simulink model "neuromodels"  (Simulink 2.20)
settings: Solver=ode45  StartTime=0.0  StopTime=999999  MaxStep=10  RelTol=1e-3  AbsTol=1e-3
values from neighbouring files (symbols this model uses):
  a = a    [buttfilt.m]
settings Model: SaveTime=off  SaveOutput=off  ConsistencyChecking=off  RTWPlaceOutputsASAP=off

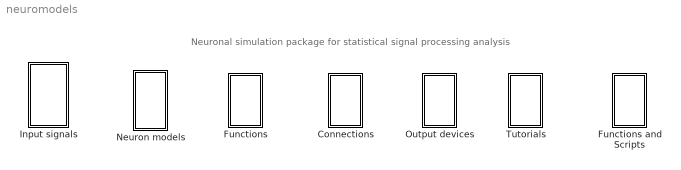
== system neuromodels ==
  note: Neuronal simulation package for statistical signal processing analysis
  Connections : Subsystem
  Functions : Subsystem
  Functions and Scripts : Subsystem
  "Input signals " : Subsystem
  Neuron models : Subsystem
  Output devices : Subsystem
  Tutorials : Subsystem

== system neuromodels/Connections ==
  note: Connection elements
  Gain : Gain  Gain=1
  Inner Product : Subsystem
      mask Type: Dot Product
      mask Description:
      | Inner (dot) product.
      | y=sum(u1.*u2)
      mask Help: Computes the inner (dot) product of the inputs: sum(u1.*u2).  The inputs are vectors of the same length. Output is a scalar.
      mask Display: disp('.\n')
  Sum : Sum  Inputs=++

== system neuromodels/Functions ==
  note: Functions
  Exponential  low-pass filter : DiscreteFilter  Numerator=k2  Denominator=1  SampleTime=dt  mask(Exponential low-pass filter){@1=20, @2=512, @3=tstep}
      mask prompts: @1 "Time constant [msec]"; @2 "Number of  points"; @3 "time step [msec]"
      mask help: Parameters
      mask init:
      | tau = @1; n = @2; dt = @3; t = [0:1:n-1]*dt; k2 = exp(-t/tau) ; k2 = k2/norm(k2);
      mask Display: plot(t,k2);
  Half-wave rectifier : Fcn  Expr=0.5*(u[1] + abs(u[1]))  mask(half-wave rectifier){}
      mask init:
      | x = [-2:0.1:2]; y = 0.5*(x+abs(x));
      mask Display: plot(x,y);
  LGN transfer function : DiscreteFilter  Numerator=k2  Denominator=1  SampleTime=dt  mask(LGN transfer function){@1=5.5, @2=tstep, @3=1500}
      mask prompts: @1 "cut-off frequency [Hz]"; @2 "time step [msec]"; @3 "time constant [msec]"
      mask help: Parameters
      mask init:
      | omega_c = @1*2*pi; dt = @2; tau = @3*1e-3; b = sqrt(omega_c^2 + tau^(-2)) ; tv = [0:dt:512]; tv_s = tv*1e-3; k2 = tv_s.*(tau + 0.5*(1-tau*b)*tv_s).*exp(-b*tv_s); k2 = k2/norm(k2);
      mask Display: plot(tv,k2);

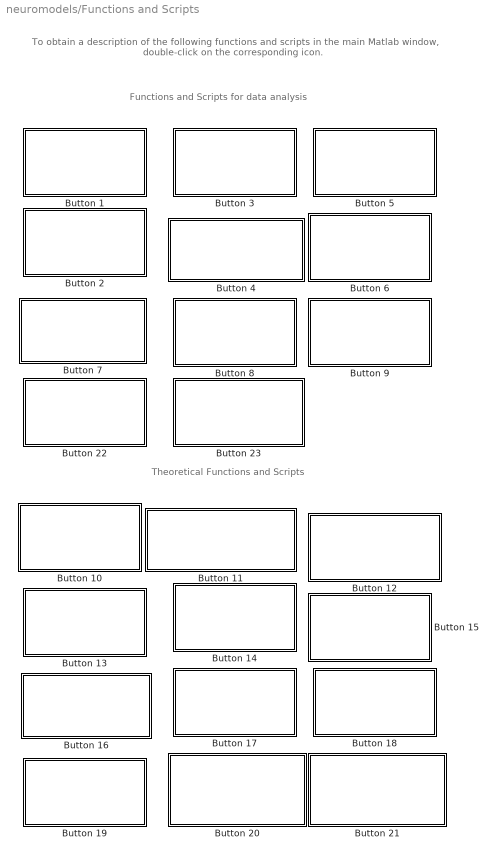
== system neuromodels/Functions and Scripts ==
  note: Functions and Scripts for data analysis
  note: To obtain a description of the following functions and scripts in
      | the main Matlab window, double-click on the corresponding icon.
  note: Theoretical Functions and Scripts
  Button 1 : Subsystem
      settings: OpenFcn=help psautostim
      mask Description: Button 1disp('End');
      mask Display: disp('Power spectrum \nand autocorrelation \nof a stimulus')
  Button 10 : Subsystem
      settings: OpenFcn=help fithifref
      mask Description: Button 10disp('End');
      mask Display: disp('F-I curve of an\nintegrate-and-fire\nneuron  ')
  Button 11 : Subsystem
      settings: OpenFcn=help fithlifref
      mask Description: Button 11disp('End');
      mask Display: disp('F-I curve of a\nleaky integrate-and-fire\nneuron ')
  Button 12 : Subsystem
      settings: OpenFcn=help gfitheor
      mask Description: Button 12disp('End');
      mask Display: disp('ISI distribution of\n random threshold \nneuron models\n(gamma and Poisson \ndistributions)  ')
  Button 13 : Subsystem
      settings: OpenFcn=help gpstheor
      mask Description: Button 13disp('End');
      mask Display: disp('Power spectrum and\nautocorrelation of\nrandom threshold\nneurons ')
  Button 14 : Subsystem
      settings: OpenFcn=help buttfilt
      mask Description: Button 14disp('End');
      mask Display: disp('Transfer function\nof a Butterworth\ndigital filter ')
  Button 15 : Subsystem
      settings: OpenFcn=help lgnfilt
      mask Description: Button 15disp('End');
      mask Display: disp('Transfer function of \na LGN thalamic\nrelay cell  ')
  Button 16 : Subsystem
      settings: OpenFcn=help poisscnt
      mask Description: Button 16disp('End');
      mask Display: disp('Count distribution for \na Poisson process ')
  Button 17 : Subsystem
      settings: OpenFcn=help neymtacnt
      mask Description: Button 17disp('End');
      mask Display: disp('Neyman type A\ncount distribution')
  Button 18 : Subsystem
      settings: OpenFcn=help prefdisp
      mask Description: Button 18disp('End');
      mask Display: disp('Variance vs. mean\ndispersion for\na Poisson process\nwith ref. period')
  Button 19 : Subsystem
      settings: OpenFcn=help sndpdisp
      mask Description: Button 19disp('End');
      mask Display: disp('Variance vs. mean\ndispersion for a\nshot noise driven\nPoisson process')
  Button 2 : Subsystem
      settings: OpenFcn=help psautospk
      mask Description: Button 2disp('End');
      mask Display: disp('Power spectrum \nand autocorrelation \nof a spike train')
  Button 20 : Subsystem
      settings: OpenFcn=help gaussroc
      mask Description: Button 20disp('End');
      mask Display: disp('ROC curves\nfor\nGaussian distributions')
  Button 21 : Subsystem
      settings: OpenFcn=help stesttheor
      mask Description: Button 21disp('End');
      mask Display: disp('Coding fraction vs. \nmean firing rate \nplot for  \nPoisson neurons')
  Button 22 : Subsystem
      settings: OpenFcn=help roc
      mask Description: Button 22disp('End');
      mask Display: disp('ROC curve \nfor two spike \ncount distributions')
  Button 23 : Subsystem
      settings: OpenFcn=help stestf
      mask Description: Button 23disp('End'); eval('help stestf1'); disp('End');
      mask Display: disp('Dependence of the \n accuracy of stimulus\n estimation on the\n mean firing rate')
  Button 3 : Subsystem
      settings: OpenFcn=help isidist
      mask Description: Button 3disp('End');
      mask Display: disp('ISI distribution\nof a spike train')
  Button 4 : Subsystem
      settings: OpenFcn=help stimest
      mask Description: Button 4disp('End');
      mask Display: disp('Estimation of a random\nstimulus from\na spike train\n(Wiener-Kolmogorov)')
  Button 5 : Subsystem
      settings: OpenFcn=help wiener1
      mask Description: Button 5disp('End');
      mask Display: disp('First order\nwiener kernel')
  Button 6 : Subsystem
      settings: OpenFcn=help countprob
      mask Description: Button 6disp('End');
      mask Display: disp('Distribution of  spike\ncounts in an\ninterval')
  Button 7 : Subsystem
      settings: OpenFcn=help dispersion
      mask Description: Button 7disp('End');
      mask Display: disp('Dispersion of the \nspike count\n(variance vs. mean)  ')
  Button 8 : Subsystem
      settings: OpenFcn=help roc
      mask Description: Button 8disp('End');
      mask Display: disp('ROC curve for\nspike count\ndistributions')
  Button 9 : Subsystem
      settings: OpenFcn=help ficurve
      mask Description: Button 9disp('End');
      mask Display: disp('Firing frequency vs. \ninjected current')

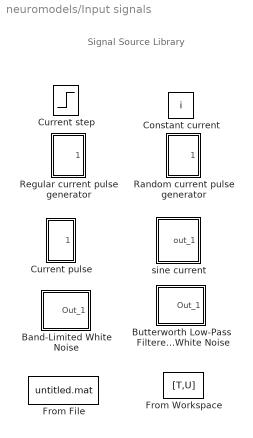
== system neuromodels/Input signals  ==
  note: Signal Source Library
  Band-Limited White Noise : Subsystem  mask(Discrete time white noise. ){@1=tstep, @2=0.1, @3=[23341]}
      mask prompts: @1 "time step [msec]"; @2 "standard deviation [nA]"; @3 "random seed"
      mask help: Discrete time white noise
      mask init:
      | dt = @1; sigma = @2; seed = @3; r = rand(1,12); r2 = [r(1),r;r,r(12)]; t =[1:13;1:13];
      mask Help: Generates a sequence of normally distributed random numbers with standard deviation sigma
      mask Display: plot(t(:),r2(:))
  Butterworth Low-Pass  Filtered White Noise : Subsystem  mask(Low-pass filtered white noise. ){@1=tstep, @2=0.63, @3=[23341], @4=240, @5=4}
      mask prompts: @1 "time step [msec]"; @2 "standard deviation [nA]"; @3 "random seed"; @4 "Cut-off frequency [Hz]"; @5 "filter order"
      mask help: Discrete time white noise
      mask init:
      | dt = @1; sigma = @2; seed = @3;[bint, a] = butter(@5,@4*2*@1*1e-3); h = freqz(bint,a); nfac = sum(h.*conj(h))/length(h); b = bint/sqrt(nfac); n = @5; x = rand(1,10*@5); y = filter(b,a,x);
      mask Help: Generates a Gaussian noise with fixed standard deviation  in the time domain and fixed cut-off frequency in the frequency domain.
      mask Display: plot((5*n:10*n),y(5*n:10*n));
  Constant current : Constant  Value=i  mask(constant current){@1=0.6}
      mask prompts: @1 "constant current value [nA]"
      mask help: Parameter
      mask init:
      | i = @1;
      mask Help: Provides a constant input current
  Current pulse : Subsystem  mask(Current step){@1=tstep, @2=100, @3=200, @4=1}
      mask prompts: @1 "time step [msec]"; @2 "start time [msec]"; @3 "pulse length [msec]"; @4 "current value [nA]"
      mask help: Parameters:
      mask init:
      | dt = @1; s = @2; w = @3; h =@4;
      mask Help: At onset tiFor a detailed description of the block, please type 'help stepc' in the main matlab window
      mask Display: plot(0,0,100,100,[10,30,30,70,70,90],[20,20,80,80,20,20])
  Current step : Step  Time=t_on  Before=i_in  After=i_fin  mask(Current step){@1=0, @2=0, @3=0}
      mask prompts: @1 "onset time [msec]"; @2 "initial current [nA]"; @3 "final current [nA]"
      mask help: Parameters
      mask init:
      | t_on = @1; i_in = @2; i_fin = @3;
      mask Help: At onset time the value of the current switches between the initial and final value
  From Workspace : FromWorkspace  VariableName=[T,U]
  From File : FromFile  FileName=untitled.mat
  Random current pulse generator : Subsystem  mask(Pulse generator){@1=tstep, @2=100, @3=20, @4=2, @5=1}
      mask prompts: @1 "time step [msec]"; @2 "start time [msec]"; @3 "period [msec]"; @4 "width [msec]"; @5 "pulse height [nA]"
      mask help: Parameters:
      mask init:
      | dt = @1; s = @2; p = @3; w = @4; h = @5;
      mask Help: Pulse generator, for a detailled description of the model, type 'help pulsegen' in the main matlab window
      mask Display: plot(0,0,100,100,[90,75,75,60,60,35,35,20,20,10],[20,20,80,80,20,20,80,80,20,20])
  Regular current pulse generator : Subsystem  mask(Pulse generator){@1=tstep, @2=100, @3=50, @4=10, @5=1}
      mask prompts: @1 "time step [msec]"; @2 "start time [msec]"; @3 "period [msec]"; @4 "width [msec]"; @5 "pulse height [nA]"
      mask help: Parameters:
      mask init:
      | dt = @1; s = @2; p = @3; w = @4; h = @5;
      mask Help: Pulse generator, for a detailled description of the model, type 'help pulsegen' in the main matlab window
      mask Display: plot(0,0,100,100,[90,75,75,60,60,35,35,20,20,10],[20,20,80,80,20,20,80,80,20,20])
  sine current : Subsystem  mask(sine current){@1=tstep, @2=2, @3=10, @4=0.25, @5=2}
      mask prompts: @1 "time step [msec]"; @2 "sine amplitude [nA]"; @3 "frequency [Hz]"; @4 "phase [percent of period]"; @5 "offset current [nA]"
      mask help: Parameters
      mask init:
      | dt = @1; a = @2; f = @3; p = @4; o = @5;
      mask Help: For detailed information about this block, please type 'help sinec' in the main matlab window
      mask Display: plot(0,-1.2,120,1.2,(0:100),sin((2*pi).*(0:100)./100))

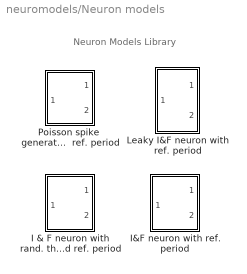
== system neuromodels/Neuron models ==
  note: Neuron Models Library
  I & F neuron with rand. thres. and ref. period : Subsystem  mask(I&F g. thres., ref. per.){@1=tstep, @2=10, @3=2, @4=0.5, @5=5}
      mask prompts: @1 "time step [msec]"; @2 "mean threshold [mV]"; @3 "gamma distr. order"; @4 "Capacitance [nF]"; @5 "refractory period [msec]"
      mask help: Parameters
      mask init:
      | dt = @1; thres = @2; n = @3; C = @4; ref = @5; if (ref<dt) disp(' '); disp('Warning: refractory period cannot be smaller than time step.'); disp(' '); end;
      mask Help: For a detailled description of the model, please type 'help giandfr' in the main matlab window
      mask Display: disp('Vm \n\n spikes')
  I&F neuron with ref. period : Subsystem  mask(I&F ref. per. ){@1=tstep, @2=10, @3=.5, @4=5}
      mask prompts: @1 "time step [msec]"; @2 "threshold [mV]"; @3 "Capacitance [nF]"; @4 "refractory period [msec]"
      mask help: Parameters
      mask init:
      | dt = @1; thres = @2; C = @3; ref = @4; if (ref<dt) disp(' '); disp('Warning: refractory period cannot be smaller than time step.'); disp(' '); end;
      mask Help: For a detailled description of the model, please type 'help iandfr' in the main matlab window
      mask Display: disp('Vm \n\n spikes')
  Leaky I&F neuron with ref. period : Subsystem  mask(L I&F ref. per.){@1=tstep, @2=10, @3=.5, @4=50, @5=5}
      mask prompts: @1 "time step [msec]"; @2 "threshold [mV]"; @3 "Capacitance [nF]"; @4 "Resistance [MOhms]"; @5 "refractory period [msec]"
      mask help: Parameters
      mask init:
      | dt = @1; thres = @2; C = @3; R = @4; ref = @5; if (ref<dt) disp(' '); disp('Warning: refractory period cannot be smaller than time step.'); disp(' '); end;
      mask Help: For a detailled description of the model, please type 'help liandfr' in the main matlab window.
      mask Display: disp('Vm \n\n spikes')
  Poisson spike  generator with  ref. period : Subsystem  mask(I&F p. thres., ref. per.){@1=tstep, @2=10, @3=.5, @4=5}
      mask prompts: @1 "time step [msec]"; @2 "mean threshold [mV]"; @3 "Capacitance [nF]"; @4 "refractory period [msec]"
      mask help: Parameters
      mask init:
      | dt = @1; thres = @2; C = @3; ref = @4; if (ref<dt) disp(' '); disp('Warning: refractory period cannot be smaller than time step.'); disp(' '); end;
      mask Help: For a detailled description of the model, please type 'help piandfr' in the main matlab window
      mask Display: disp('Vm \n\n spikes')

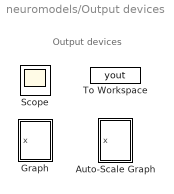
== system neuromodels/Output devices ==
  note: Output devices
  Auto-Scale Graph : Subsystem  mask(Storage scope.){@1=5, @2=-10, @3=10, @4=200, @5='y-/g--/c-./w:/m*/ro/b+'}
      mask prompts: @1 "Initial Time Range:"; @2 "Initial y-min:"; @3 "Initial y-max:"; @4 "Storage pts.:"; @5 "Line type (rgbw-.:xo):"
      mask help:
      | Storage scope using MATLAB graph window.
      | Enter plotting ranges and line type.
      mask init:
      | npts = @4; color = @5; ax = [0, @1, @2, @3]; dt=-1;
      mask Help: This block uses a MATLAB figure window to plot the input signal.  The graph limits are automatically scaled to the min and max values of the signal stored in the scope's signal buffer.  Line type must be in quotes.  See the M-file sfunyst.m.
      mask Display: plot(0,0,100,100,[83,76,63,52,42,38,28,16,11,84,11,11,11,90,90,11],[75,58,47,54,72,80,84,74,65,65,65,90,40,40,90,90])
  Graph : Subsystem  mask(Graph scope.){@1=20, @2=-1.1, @3=1.2, @4='y-/g--/c-./w:/m*/ro/b+'}
      mask prompts: @1 "Time range:"; @2 "y-min:"; @3 "y-max:"; @4 "Line type (rgbw-:*). Seperate each plot by '/':"
      mask help:
      | Graph scope using MATLAB graph window.
      | Enter plotting ranges and line type.
      mask init:
      | color = @4; ax = [0, @1, @2, @3]; dt = -1;
      mask Help: This block plots to the MATLAB graph window and can be used as an improved version of the Scope block. Look at the m-file sfuny.m to see how it works. This block can take scalar or vector input signal.
      mask Display: plot(0,0,100,100,[90,10,10,10,90,90,10],[65,65,90,40,40,90,90],[90,78,69,54,40,31,25,10],[77,60,48,46,56,75,81,84])
  Scope : Scope
      settings: TickLabels=on  TimeRange=1.000000  YMin=-1.000000  YMax=1.000000  SaveToWorkspace=off  SaveName=ScopeData
  To Workspace : ToWorkspace  VariableName=yout  SampleTime=0
      settings: Buffer=1000

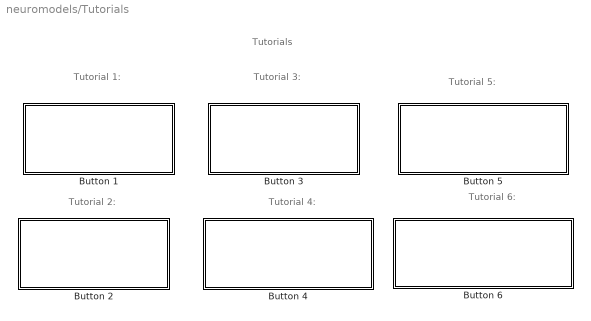
== system neuromodels/Tutorials ==
  note: Tutorials
  note: Tutorial 1:
  note: Tutorial 4:
  note: Tutorial 2:
  note: Tutorial 6:
  note: Tutorial 3:
  note: Tutorial 5:
  Button 1 : Subsystem
      settings: OpenFcn=tutorial1prep
      mask Display: disp('ISI distribution,\nPower spectrum\nand\nAutocorrelation function')
  Button 2 : Subsystem
      settings: OpenFcn=tutorial2prep
      mask Display: disp('FI-curve of a \nleaky integrate \nand fire neuron')
  Button 3 : Subsystem
      settings: OpenFcn=tutorial3prep
      mask Display: disp('Estimation of a random\nstimulus encoded in\na Poisson spike train')
  Button 4 : Subsystem
      settings: OpenFcn=tutorial4prep
      mask Display: disp('Estimation of the\ntransfer function of a\nneuron model\n(first order Wiener kernel)')
  Button 5 : Subsystem
      settings: OpenFcn=tutorial5prep
      mask Display: disp('Multiplicative and refractory\neffects in a model\nof retinal ganglion cells')
  Button 6 : Subsystem
      settings: OpenFcn=tutorial6prep
      mask Display: disp('Dependence of the accuracy\nof stimulus encoding\non the mean firng rate of\nPoisson neurons')

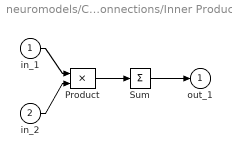
== system neuromodels/Connections/Inner Product ==
  in_1 : Inport  Port=1  PortWidth=-1  SampleTime=-1
  in_2 : Inport  Port=2  PortWidth=-1  SampleTime=-1
  Product : Product  Inputs=2
  Sum : Sum  Inputs=+
  out_1 : Outport  Port=1  InitialOutput=0
  wires:
  in_2/1 -> Product/2
  in_1/1 -> Product/1
  Product/1 -> Sum/1
  Sum/1 -> out_1/1

== system neuromodels/Functions and Scripts/Button 1 ==

== system neuromodels/Functions and Scripts/Button 10 ==

== system neuromodels/Functions and Scripts/Button 11 ==

== system neuromodels/Functions and Scripts/Button 12 ==

== system neuromodels/Functions and Scripts/Button 13 ==

== system neuromodels/Functions and Scripts/Button 14 ==

== system neuromodels/Functions and Scripts/Button 15 ==

== system neuromodels/Functions and Scripts/Button 16 ==

== system neuromodels/Functions and Scripts/Button 17 ==

== system neuromodels/Functions and Scripts/Button 18 ==

== system neuromodels/Functions and Scripts/Button 19 ==

== system neuromodels/Functions and Scripts/Button 2 ==

== system neuromodels/Functions and Scripts/Button 20 ==

== system neuromodels/Functions and Scripts/Button 21 ==

== system neuromodels/Functions and Scripts/Button 22 ==

== system neuromodels/Functions and Scripts/Button 23 ==

== system neuromodels/Functions and Scripts/Button 3 ==

== system neuromodels/Functions and Scripts/Button 4 ==

== system neuromodels/Functions and Scripts/Button 5 ==

== system neuromodels/Functions and Scripts/Button 6 ==

== system neuromodels/Functions and Scripts/Button 7 ==

== system neuromodels/Functions and Scripts/Button 8 ==

== system neuromodels/Functions and Scripts/Button 9 ==

== system neuromodels/Input signals /Band-Limited White Noise ==
  Gain : Gain  Gain=sigma
  White Noise : RandomNumber  Mean=0  Variance=1  Seed=seed  SampleTime=-1
  Zero-Order Hold : ZeroOrderHold  SampleTime=dt
  Out_1 : Outport  Port=1  InitialOutput=0
  wires:
  White Noise/1 -> Zero-Order Hold/1
  Gain/1 -> Out_1/1
  Zero-Order Hold/1 -> Gain/1

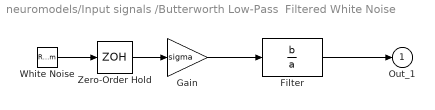
== system neuromodels/Input signals /Butterworth Low-Pass  Filtered White Noise ==
  Filter : DiscreteFilter  Numerator=b  Denominator=a  SampleTime=dt
  Gain : Gain  Gain=sigma
  White Noise : RandomNumber  Mean=0  Variance=1  Seed=seed  SampleTime=-1
  Zero-Order Hold : ZeroOrderHold  SampleTime=dt
  Out_1 : Outport  Port=1  InitialOutput=0
  wires:
  Gain/1 -> Filter/1
  Filter/1 -> Out_1/1
  White Noise/1 -> Zero-Order Hold/1
  Zero-Order Hold/1 -> Gain/1

== system neuromodels/Input signals /Current pulse ==
  Current step : S-Function  FunctionName=stepc  Parameters="dt, s,  w, h"  PortCounts=[]  SFunctionModules=''
  out_1 : Outport  Port=1  InitialOutput=0
  wires:
  Current step/1 -> out_1/1

== system neuromodels/Input signals /Random current pulse generator ==
  Random current pulse generator : S-Function  FunctionName=ppulsegen  Parameters=dt,s,p,w,h  PortCounts=[]  SFunctionModules=''
  out_1 : Outport  Port=1  InitialOutput=0
  wires:
  Random current pulse generator/1 -> out_1/1

== system neuromodels/Input signals /Regular current pulse generator ==
  Regular current pulse generator : S-Function  FunctionName=pulsegen  Parameters=dt,s,p,w,h  PortCounts=[]  SFunctionModules=''
  out_1 : Outport  Port=1  InitialOutput=0
  wires:
  Regular current pulse generator/1 -> out_1/1

== system neuromodels/Input signals /sine current ==
  S-Function2 : S-Function  FunctionName=sinec  Parameters=dt,a,f,p,o  PortCounts=[]  SFunctionModules=''
  out_1 : Outport  Port=1  InitialOutput=0
  wires:
  S-Function2/1 -> out_1/1

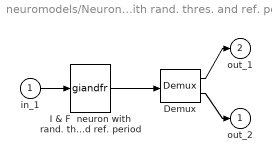
== system neuromodels/Neuron models/I & F neuron with rand. thres. and ref. period ==
  in_1 : Inport  Port=1  PortWidth=-1  SampleTime=-1
  Demux : Demux  Outputs=2
  I & F  neuron with rand. thres. and ref. period : S-Function  FunctionName=giandfr  Parameters=dt,thres,n,C,ref  PortCounts=[]  SFunctionModules=''
  out_2 : Outport  Port=1  InitialOutput=0
  out_1 : Outport  Port=2  InitialOutput=0
  wires:
  in_1/1 -> I & F  neuron with rand. thres. and ref. period/1
  Demux/2 -> out_2/1
  Demux/1 -> out_1/1
  I & F  neuron with rand. thres. and ref. period/1 -> Demux/1

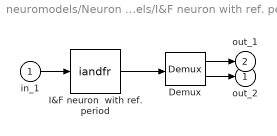
== system neuromodels/Neuron models/I&F neuron with ref. period ==
  in_1 : Inport  Port=1  PortWidth=-1  SampleTime=-1
  Demux : Demux  Outputs=2
  I&F neuron  with ref. period : S-Function  FunctionName=iandfr  Parameters=dt,thres,C,ref  PortCounts=[]  SFunctionModules=''
  out_2 : Outport  Port=1  InitialOutput=0
  out_1 : Outport  Port=2  InitialOutput=0
  wires:
  in_1/1 -> I&F neuron  with ref. period/1
  Demux/2 -> out_2/1
  Demux/1 -> out_1/1
  I&F neuron  with ref. period/1 -> Demux/1

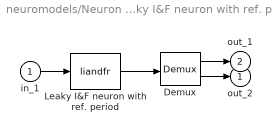
== system neuromodels/Neuron models/Leaky I&F neuron with ref. period ==
  in_1 : Inport  Port=1  PortWidth=-1  SampleTime=-1
  Demux : Demux  Outputs=2
  Leaky I&F neuron with ref. period : S-Function  FunctionName=liandfr  Parameters=dt,thres,C,R,ref  PortCounts=[]  SFunctionModules=''
  out_2 : Outport  Port=1  InitialOutput=0
  out_1 : Outport  Port=2  InitialOutput=0
  wires:
  in_1/1 -> Leaky I&F neuron with ref. period/1
  Demux/2 -> out_2/1
  Demux/1 -> out_1/1
  Leaky I&F neuron with ref. period/1 -> Demux/1

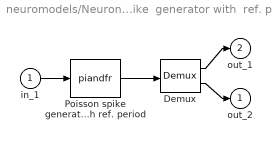
== system neuromodels/Neuron models/Poisson spike  generator with  ref. period ==
  in_1 : Inport  Port=1  PortWidth=-1  SampleTime=-1
  Demux : Demux  Outputs=2
  Poisson spike generator with ref. period : S-Function  FunctionName=piandfr  Parameters=dt,thres,C, ref  PortCounts=[]  SFunctionModules=''
  out_2 : Outport  Port=1  InitialOutput=0
  out_1 : Outport  Port=2  InitialOutput=0
  wires:
  in_1/1 -> Poisson spike generator with ref. period/1
  Demux/2 -> out_2/1
  Demux/1 -> out_1/1
  Poisson spike generator with ref. period/1 -> Demux/1

== system neuromodels/Output devices/Auto-Scale Graph ==
  x : Inport  Port=1  PortWidth=-1  SampleTime=-1
  "S-function M-file which plots lines " : S-Function  FunctionName=sfunyst  Parameters=ax, color, npts, dt  PortCounts=[]  SFunctionModules=''
  wires:
  x/1 -> "S-function M-file which plots lines "/1

== system neuromodels/Output devices/Graph ==
  x : Inport  Port=1  PortWidth=-1  SampleTime=-1
  "S-function M-file which plots lines " : S-Function  FunctionName=sfuny  Parameters=ax, color,dt  PortCounts=[]  SFunctionModules=''
  wires:
  x/1 -> "S-function M-file which plots lines "/1

== system neuromodels/Tutorials/Button 1 ==

== system neuromodels/Tutorials/Button 2 ==

== system neuromodels/Tutorials/Button 3 ==

== system neuromodels/Tutorials/Button 4 ==

== system neuromodels/Tutorials/Button 5 ==

== system neuromodels/Tutorials/Button 6 ==
